simulink model "IC_Module"  (R2024b)
settings: Solver=VariableStepAuto  StartTime=0.0  StopTime=10.0  RelTol=1e-3
values from neighbouring files (symbols this model uses):
  D_delta = 0.001    [config.m]
libraries: simulink x1
settings Model: Creator=LiHaoh  LastModifiedBy=LiHaoh

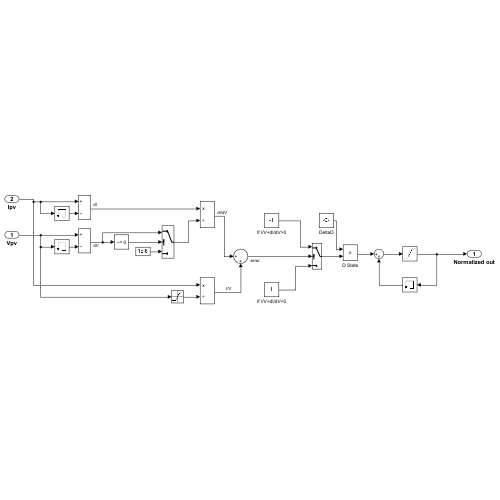
[thumbnail: Simulink's stored preview of the top-level diagram]
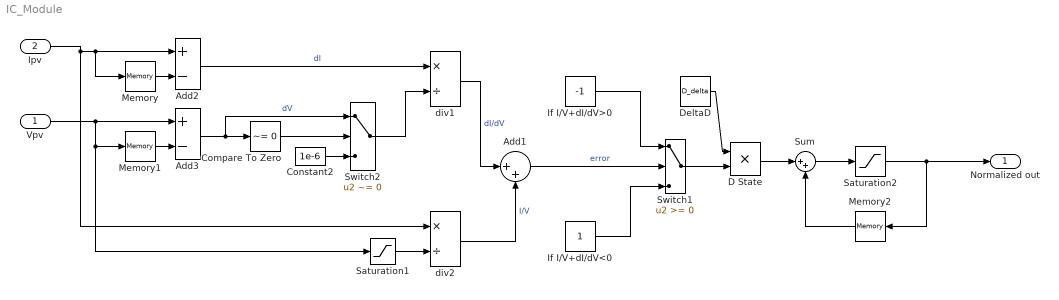
== system IC_Module ==
  Vpv : Inport
  Ipv : Inport  Port=2
  Add1 : Sum  Inputs=|++
  Add2 : Sum  Inputs=+-
  Add3 : Sum  Inputs=+-
  Compare To Zero : simulink/Logic and Bit Operations/Compare To Zero  relop=~=  OutDataTypeStr=uint8
  Constant2 : Constant  Value=1e-6
  D State : Product  RndMeth=Zero
  DeltaD : Constant  Value=D_delta
  If I/V+dI/dV<0 : Constant
  If I/V+dI/dV>0 : Constant  Value=-1
  Memory : Memory
  Memory1 : Memory
  Memory2 : Memory  InheritSampleTime=on
  Saturation1 : Saturate  UpperLimit=inf  LowerLimit=eps
  Saturation2 : Saturate  UpperLimit=0.95  LowerLimit=0.1
  Sum : Sum  Inputs=|++
  Switch1 : Switch  SaturateOnIntegerOverflow=off  InputSameDT=off
  Switch2 : Switch  Criteria=u2 ~= 0  SaturateOnIntegerOverflow=off  InputSameDT=off
  div1 : Product  Inputs=*/  RndMeth=Zero
  div2 : Product  Inputs=*/  RndMeth=Zero
  Normalized out : Outport
  wires:
  Ipv/1 -> Memory/1, Add2/1, div2/1
  DeltaD/1 -> D State/1
  Memory1/1 -> Add3/2
  If I/V+dI/dV>0/1 -> Switch1/1
  D State/1 -> Sum/1
  Add2/1 -> div1/1  "dI"
  Saturation1/1 -> div2/2
  Memory2/1 -> Sum/2
  Switch2/1 -> div1/2
  Memory/1 -> Add2/2
  If I/V+dI/dV<0/1 -> Switch1/3
  div2/1 -> Add1/2  "I/V"
  Vpv/1 -> Add3/1, Memory1/1, Saturation1/1
  Add3/1 -> Compare To Zero/1, Switch2/1  "dV"
  Sum/1 -> Saturation2/1
  Constant2/1 -> Switch2/3
  Switch1/1 -> D State/2
  Compare To Zero/1 -> Switch2/2
  Add1/1 -> Switch1/2  "error"
  div1/1 -> Add1/1  "dI/dV"
  Saturation2/1 -> Normalized out/1, Memory2/1
